simulink library "bcm"  (R2021b)
settings: Solver=VariableStepAuto  StartTime=0.0  StopTime=10.0  RelTol=1e-3
undefined symbols (not defined in the file or in its folder): ENUM_ANTITHEFT_ALARM, ENUM_ANTITHEFT_ARM, ENUM_ANTITHEFT_DISARM, ENUM_ANTITHEFT_WAIT, ENUM_GEARPOSNTOCAN_P, ENUM_PDKEYRAWLULOCK_INUNLOCK, ENUM_PDKEYRAWPS_INPS, ENUM_POWERSTA_ON, ENUM_POWERSTA_READY, ENUM_POWERSTA_STANDBY, FALSE, KBCM_ALMBrightnessDark_enum, KBCM_AmbBlue_enum, KBCM_AmbBreathT_ms, KBCM_AmbGreen_enum, KBCM_AmbRed_enum, KBCM_Antitheft_enum_ovrdflg, KBCM_Antitheft_enum_ovrdval, KBCM_APMDoorCtrlSta_flg_ovrdflg, KBCM_APMDoorCtrlSta_flg_ovrdval, KBCM_DelayTSW_flg, KBCM_DiagFLTC_mA, KBCM_DiagFMHT_s, KBCM_DiagFRTC_mA, KBCM_DiagRLTC_mA, KBCM_DiagRRTC_mA, KBCM_DrAPMRetryTimes_cnt, KBCM_DrOpenWdwOT_s, KBCM_DrOpenWdwReady_s, KBCM_ESSOffT_ms, KBCM_ESSOnT_ms, KBCM_IVIRstHoldT_ms, KBCM_IVIRstTriggerT_ms, KBCM_ONDelayT_ms, KBCM_ReDetectT_K, KBCM_RmLampKeep_min, KBCM_RmLpKeyInT_s, KBCM_RmLpKeyMissT_s, KBCM_SlpDebounceTime_s, KBCM_SPTGDetectT_sec, KBCM_SPTGLeave_flg, KBCM_SPTGLeftBound_cm, KBCM_SPTGLeftBoundOut_cm, KBCM_SPTGLowerBound_cm, KBCM_SPTGLowerBoundOut_cm, KBCM_SPTGRightBound_cm, KBCM_SPTGRightBoundOut_cm, KBCM_SPTGTOut_K, KBCM_SPTGUpperBound_cm, KBCM_SPTGUpperBoundOut_cm, KBCM_SPTGWaitDKC_sec, KBCM_TrunSWKeepTime3_s, KBCM_TrunSWKeepTime5_s, KBCM_TrunSWKeepTime7_s, KBCM_USSDis_cm, KBCM_USSFilterT_K, KBCM_WaitAPMPwr_K, KBCM_WdwManualDetT_s, MIN2SEC, TRUE ... (+1)
libraries: simulink x151, hcu_lib x5
(part 2 of 8)

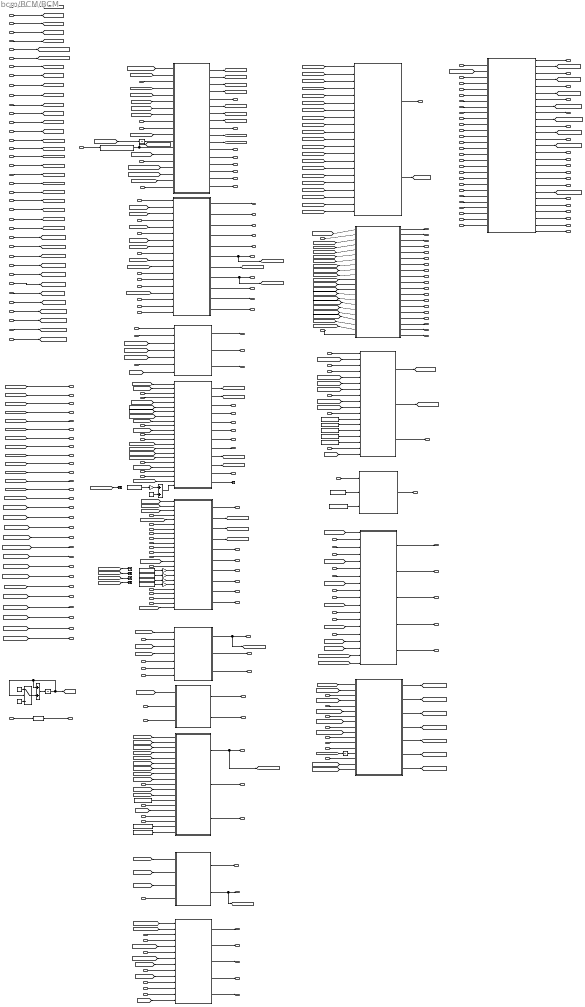
== system bcm/BCM/BCM ==
  task_time_s : Inport
  VINP_VehSpeed_kph : Inport  Port=2
  VINP_AirBagFailCmd_flg : Inport  Port=3
  VINP_ActBrkLampSta_flg : Inport  Port=4
  VINP_ESSActive_flg : Inport  Port=5
  VINP_SASAngle_Deg : Inport  Port=6
  VINP_SRRODAWarnR_enum : Inport  Port=7
  VINP_SRRODAWarnL_enum : Inport  Port=8
  VINP_SRRBSDWarnR_enum : Inport  Port=9
  VINP_SRRBSDWarnL_enum : Inport  Port=10
  VINP_LeftTurnReq_flg : Inport  Port=11
  VINP_RightTurnReq_flg : Inport  Port=12
  VINP_ForceLowBeam_enum : Inport  Port=13
  VINP_HazardWarningReq_flg : Inport  Port=14
  VINP_SetUnlockSingle_flg : Inport  Port=15
  VINP_IVIStatus_flg : Inport  Port=16
  VINP_IVINightModeSta_flg : Inport  Port=17
  VINP_HeadLampSW_enum : Inport  Port=18
  VINP_RFogLampSW_flg : Inport  Port=19
  VINP_FollowMeSW_flg : Inport  Port=20
  VINP_IVIRRDefReq_flg : Inport  Port=21
  VINP_IVIWIMAINSW_flg : Inport  Port=22
  VINP_CANMsgValidIVI2_flg : Inport  Port=23
  VINP_CDLUnlockButt_flg : Inport  Port=24  OutDataTypeStr=boolean
  VINP_CDLLockButt_flg : Inport  Port=25  OutDataTypeStr=boolean
  VINP_RoomLampMode_flg : Inport  Port=26
  VINP_MFRDNBrightReq_pct : Inport  Port=27
  VINP_METERKPHCalcu_kph : Inport  Port=28
  VINP_IVIPWModeReq_enum : Inport  Port=29
  VINP_AmbLighLowBatAlertSW_flg : Inport  Port=30
  VINP_AmbLighSafetyAlertSW_flg : Inport  Port=31
  VINP_AmbLightBrightnessSet_enum : Inport  Port=32
  VINP_AmbLightDimInDarkSW_flg : Inport  Port=33
  VINP_AmbLightSW_flg : Inport  Port=34
  VINP_AmbLightWlcmLightSW_flg : Inport  Port=35
  VINP_LINKtoDRIVE_flg : Inport  Port=36
  VINP_AmbLightColorSet_enum : Inport  Port=37
  VINP_IVIPTGUSStaSW_flg : Inport  Port=38
  VINP_LDrvControlCommand_pct : Inport  Port=39
  VINP_LPasControlCommand_pct : Inport  Port=40
  VINP_LRLDControlCommand_pct : Inport  Port=41
  VINP_LRRDControlCommand_pct : Inport  Port=42
  VINP_OpenDrOpenWdoSW_flg : Inport  Port=43
  VINP_CANMsgValidIVI1_flg : Inport  Port=44
  VINP_UserSet_enum : Inport  Port=45
  VINP_TurnSwTimeSet_enum : Inport  Port=46
  VINP_IVILockSoundSWSta_flg : Inport  Port=47
  VINP_AVMparkingmode_enum : Inport  Port=48
  VINP_HVBattSOCDis_pct : Inport  Port=49
  VINP_CSW2DimSwSta_flg : Inport  Port=50
  VINP_CSW2PassSWSta_flg : Inport  Port=51
  VINP_CSW2FWipSwSta_enum : Inport  Port=52
  VINP_CSW2FWasSwSta_enum : Inport  Port=53
  VUNP_CSW2TurnSwSta_enum : Inport  Port=54
  VINP_CSW2RWipWasSwSta_enum : Inport  Port=55
  VINP_PCommandToBCM_enum : Inport  Port=56
  VINP_DrLockSta_flg : Inport  Port=57
  VINP_CSWDimSw_flg : Inport  Port=58
  VINP_CSWPassSWSta_flg : Inport  Port=59
  VINP_RLSLampSta_flg : Inport  Port=60
  VINP_CSWTurnSWSta_enum : Inport  Port=61
  VINP_RLTurnLampC_mA : Inport  Port=62
  VINP_RRTurnLampC_mA : Inport  Port=63
  VINP_FLTurnLampC_mA : Inport  Port=64
  VINP_FRTurnLampC_mA : Inport  Port=65
  VINP_MIRRORFOLDSW_flg : Inport  Port=66
  VINP_CSWFWasSWSta_enum : Inport  Port=67
  VINP_CSWFWipSWSta_enum : Inport  Port=68
  VINP_RLSRainSnrWiperCmd_enum : Inport  Port=69
  VINP_FWiperAS_flg : Inport  Port=70
  VINP_CSWRWipIntSwSta_enum : Inport  Port=71
  VINP_RWiperAS_flg : Inport  Port=72
  VINP_CSWRWasSWSta_enum : Inport  Port=73
  VINP_PTGRDILsta_enum : Inport  Port=74
  VINP_RWiperProtection_flg : Inport  Port=75
  VINP_FWiperProtection_flg : Inport  Port=76
  VINP_PDKeyAreaPTG_enum : Inport  Port=77
  VINP_SWCmodeSta_flg : Inport  Port=78
  VINP_CANMsgValidDKC1_flg : Inport  Port=79
  VINP_CANMsgValidGWZoneDR1_flg : Inport  Port=80
  VINP_CANMsgValidGWZoneFR1_flg : Inport  Port=81
  VINP_PTGInnerSW2_enum : Inport  Port=82
  VINP_LDrvValWdwOpened_pct : Inport  Port=83
  VINP_LPasValWdwOpened_pct : Inport  Port=84
  VINP_LRLDValWdwOpened_pct : Inport  Port=85
  VINP_LRRDValWdwOpened_pct : Inport  Port=86
  VINP_PDKeyAreaLockUnlock_enum : Inport  Port=87
  VINP_PDKeyAreaPS_enum : Inport  Port=88
  VINP_ReDoorLock_enum : Inport  Port=89
  VINP_ReOutsideMirror_enum : Inport  Port=90
  VINP_HoodSW_flg : Inport  Port=91
  VINP_TailgateSW_flg : Inport  Port=92
  VINP_DrDoorSW_flg : Inport  Port=93
  VINP_PsDoorSW_flg : Inport  Port=94
  VINP_RLDoorSW_flg : Inport  Port=95
  VINP_RRDoorSW_flg : Inport  Port=96
  VINP_TrunkHanSW_flg : Inport  Port=97
  VINP_HazardSW_flg : Inport  Port=98
  VINP_CentralDoorLockSW_flg : Inport  Port=99
  VINP_BrakeSWGPIO_flg : Inport  Port=100
  VPMM_PwrSta_enum : Inport  Port=101
  VTQD_ShiftGearPosn_enum : Inport  Port=102
  VTQD_CrashDetd_flg : Inport  Port=103
  VTQD_DiagHCrash_flg : Inport  Port=104
  VTQD_ReBrakeLPReq_flg : Inport  Port=105
  VINP_FlashAntitheft_enum : Inport  Port=106
  VINP_FlashCountAlarm_enum : Inport  Port=107
  VINP_FlashMFSWTri_flg : Inport  Port=108
  VINP_FlashMirrorFlodPos : Inport  Port=109
  VINP_FlashFuelDoorPos : Inport  Port=110
  VINP_FlashLockSetting_flg : Inport  Port=111
  VINP_FlashMFRDNBrightReq_pct : Inport  Port=112
  VINP_FlashRoomLampMode_flg : Inport  Port=113
  VINP_FlashWiperFixMode_flg : Inport  Port=114
  VINP_FlashIVIPTGUSStaSW_flg : Inport  Port=115
  VINP_FlashHoodSW_flg : Inport  Port=116
  VINP_FlashTailgateSW_flg : Inport  Port=117
  VINP_FlashCTDLockSW_flg : Inport  Port=118
  VINP_FlashTailgateHDSW_flg : Inport  Port=119
  VINP_FlashAPMDoorControlSta_flg : Inport  Port=120
  VINP_FlashfUnlockSingle_flg : Inport  Port=121
  VINP_FlashAmbFunEN_enum : Inport  Port=122
  VINP_FlashAmbWelEN_enum : Inport  Port=123
  VINP_FlashAmbDimEN_enum : Inport  Port=124
  VINP_FlashAmbLinkDriSta_enum : Inport  Port=125
  VINP_FlashAmbPwrWarnEN_enum : Inport  Port=126
  VINP_FlashAmbODAEN_enum : Inport  Port=127
  VINP_FlashAmbColorSta1_enum : Inport  Port=128
  VINP_FlashAmbColorSta2_enum : Inport  Port=129
  VINP_FlashAmbColorSta3_enum : Inport  Port=130
  VINP_FlashAmbColorSta4_enum : Inport  Port=131
  VINP_FlashAmbColorSta5_enum : Inport  Port=132
  VINP_FlashAmbColorSta7_enum : Inport  Port=133
  VINP_FlashAmbBrightnessSta1_enum : Inport  Port=134
  VINP_FlashAmbBrightnessSta2_enum : Inport  Port=135
  VINP_FlashAmbBrightnessSta3_enum : Inport  Port=136
  VINP_FlashAmbBrightnessSta4_enum : Inport  Port=137
  VINP_FlashAmbBrightnessSta5_enum : Inport  Port=138
  VINP_FlashAmbBrightnessSta7_enum : Inport  Port=139
  VINP_funAuto_flg : Inport  Port=140
  VINP_DiagDRLOFF_flg : Inport  Port=141
  VINP_DiagFMHT_s : Inport  Port=142
  VINP_DiagFLTC_mA : Inport  Port=143
  VINP_DiagFRTC_mA : Inport  Port=144
  VINP_DiagRLTC_mA : Inport  Port=145
  VINP_DiagRRTC_mA : Inport  Port=146
  VAPM_PASDRMR_cm : Inport  Port=147
  VAPM_PASDRML_cm : Inport  Port=148
  VINP_APSActive_flg : Inport  Port=149
  VINP_RRDefSta_flg : Inport  Port=150
  VDDM_HVRlyOpCFS_flg : Inport  Port=151
  VDDM_MCUActCFS_flg : Inport  Port=152
  APM_Door : Subsystem
  Add1 : Sum
  Amb : Subsystem
  AntiTheft : Subsystem
  BCM_WAKE_MODULE : Subsystem
  CSW : Subsystem
  CenterDoorLock : Subsystem
  Constant10 : Constant  Value=KBCM_DelayTSW_flg
  Constant11 : Constant  Value=KBCM_ReDetectT_K
  Constant12 : Constant  Value=KBCM_SPTGDetectT_sec
  Constant13 : Constant  Value=KBCM_SPTGLeave_flg
  Constant14 : Constant  Value=KBCM_RmLampKeep_min
  Constant15 : Constant  Value=KBCM_SPTGWaitDKC_sec
  Constant16 : Constant  Value=0
  Constant17 : Constant
  Constant18 : Constant  Value=KBCM_RmLpKeyInT_s
  Constant19 : Constant  Value=KBCM_RmLpKeyMissT_s
  Constant44 : Constant  Value=KBCM_DiagFMHT_s
  Constant45 : Constant  Value=10
  Constant46 : Constant  Value=KBCM_DiagFLTC_mA
  Constant47 : Constant  Value=KBCM_DiagFRTC_mA
  Constant48 : Constant  Value=KBCM_DiagRLTC_mA
  Constant49 : Constant  Value=KBCM_DiagRRTC_mA
  Constant8 : Constant  Value=KBCM_IVIRstHoldT_ms
  Constant9 : Constant  Value=KBCM_IVIRstTriggerT_ms
  Data Type Conversion : DataTypeConversion  OutDataTypeStr=uint8
  Dimmer : Subsystem
  ExteriorLight : Subsystem
  FlasherSignal : Subsystem
  Gain{,2..4} (4 alike) : Gain  Gain=10
  Gain1 : Gain  Gain=5
  IVI Reset : Subsystem
  PTG : Subsystem
  Personal_Setting : Subsystem
  PowerMirror : Subsystem
  RearDefogger : Subsystem
  RoomLamp : Subsystem
  Sum : Sum
  Switch : Switch  Criteria=u2 > Threshold
  Tailgate : Subsystem
  Terminator{,1..5} (6 alike) : Terminator
  Unit Delay : UnitDelay  SampleTime=-1  HasFrameUpgradeWarning=on
  Unit Delay1 : UnitDelay  SampleTime=-1  HasFrameUpgradeWarning=on
  Unit Delay2 : UnitDelay  SampleTime=-1  HasFrameUpgradeWarning=on
  Verify : Subsystem
  WasherWiper : Subsystem
  VBCM_AntitheftSta_enum : Outport
  VBCM_TailgateRemote_enum : Outport  Port=2
  VBCM_HornCtrl_flg : Outport  Port=3
  VBCM_AllDoorSW_flg : Outport  Port=4
  VBCM_BCMDoorLockSta_flg : Outport  Port=5
  VBCM_AntitheftSeatFlod_flg : Outport  Port=6
  VBCM_HoodSW_flg : Outport  Port=7
  VBCM_TailgateSW_flg : Outport  Port=8
  VBCM_DrDoorSW_flg : Outport  Port=9
  VBCM_PsDoorSW_flg : Outport  Port=10
  VBCM_RLDoorSW_flg : Outport  Port=11
  VBCM_RRDoorSW_flg : Outport  Port=12
  VBCM_LockSetting_flg : Outport  Port=13
  VBCM_FrChargingDoorCtrl_enum : Outport  Port=14
  VBCM_RrChargingDoorCtrl_enum : Outport  Port=15
  VBCM_CrashSDetd_flg : Outport  Port=16
  VBCM_CTDCtrl_enum : Outport  Port=17
  VBCM_DoorLockIND_flg : Outport  Port=18
  VBCM_CTDLockSW_flg : Outport  Port=19
  VBCM_Dimmer_pct : Outport  Port=20
  VBCM_DimmerEN_flg : Outport  Port=21
  VBCM_PosLamp_flg : Outport  Port=22
  VBCM_LBeam_flg : Outport  Port=23
  VBCM_HBeam_flg : Outport  Port=24
  VBCM_RrFogLamp_flg : Outport  Port=25
  VBCM_BrakeLamp_flg : Outport  Port=26
  VBCM_ReverseLamp_flg : Outport  Port=27
  VBCM_LDRL_flg : Outport  Port=28
  VBCM_RDRL_flg : Outport  Port=29
  VBCM_LBSD_flg : Outport  Port=30
  VBCM_RBSD_flg : Outport  Port=31
  VBCM_HazardSW_flg : Outport  Port=32
  VBCM_LTurnLP_flg : Outport  Port=33
  VBCM_RTurnLP_flg : Outport  Port=34
  VBCM_BCMBuzzerReq_flg : Outport  Port=35
  VBCM_MirrorCtrl_enum : Outport  Port=36
  VBCM_MirrorDefog_flg : Outport  Port=37
  VBCM_RrDefog_flg : Outport  Port=38
  VBCM_RoomLampH_flg : Outport  Port=39
  VBCM_RoomLampL_flg : Outport  Port=40
  VBCM_TrunkRel_flg : Outport  Port=41
  VBCM_TailgateHDSW_flg : Outport  Port=42
  VBCM_FWiperL_flg : Outport  Port=43
  VBCM_FWiperH_flg : Outport  Port=44
  VBCM_RWiper_flg : Outport  Port=45
  VBCM_WasherCtrl_enum : Outport  Port=46
  VBCM_WiperFixMode_flg : Outport  Port=47
  VBCM_SleepReq_flg : Outport  Port=48
  VBCM_AmbLightBreath1_enum : Outport  Port=49
  VBCM_AmbLightBreath2_enum : Outport  Port=50
  VBCM_AmbLightBreath3_enum : Outport  Port=51
  VBCM_AmbLightBreath4_enum : Outport  Port=52
  VBCM_AmbLightBreath5_enum : Outport  Port=53
  VBCM_AmbLightBreath6_enum : Outport  Port=54
  VBCM_AmbLightBrightness1_enum : Outport  Port=55
  VBCM_AmbLightBrightness2_enum : Outport  Port=56
  VBCM_AmbLightBrightness3_enum : Outport  Port=57
  VBCM_AmbLightBrightness4_enum : Outport  Port=58
  VBCM_AmbLightBrightness5_enum : Outport  Port=59
  VBCM_AmbLightBrightness6_enum : Outport  Port=60
  VBCM_AmbLightColor1_enum : Outport  Port=61
  VBCM_AmbLightColor2_enum : Outport  Port=62
  VBCM_AmbLightColor3_enum : Outport  Port=63
  VBCM_AmbLightColor4_enum : Outport  Port=64
  VBCM_AmbLightColor5_enum : Outport  Port=65
  VBCM_AmbLightColor6_enum : Outport  Port=66
  VBCM_LampPwr_flg : Outport  Port=67
  VBCM_SPTGDet_flg : Outport  Port=68
  VBCM_APSOpenPTG_flg : Outport  Port=69
  VBCM_FollowMe_flg : Outport  Port=70
  VBCM_IVIRST_flg : Outport  Port=71
  VBCM_CountAlarm_enum : Outport  Port=72
  VBCM_MFSWTri_flg : Outport  Port=73
  VBCM_MirrorFlodPos_flg : Outport  Port=74
  VBCM_FuelDoorPos_flg : Outport  Port=75
  VBCM_MFRDNBrightReq_pct : Outport  Port=76
  VBCM_RoomLampMode_flg : Outport  Port=77
  VBCM_IVIPTGUSStaSW_flg : Outport  Port=78
  VBCM_PTGInnerSW2_enum : Outport  Port=79
  VBCM_DiagHCrash_flg : Outport  Port=80
  VBCM_DiagFLTS_flg : Outport  Port=81
  VBCM_DiagFRTS_flg : Outport  Port=82
  VBCM_DiagRLTS_flg : Outport  Port=83
  VBCM_DiagRRTS_flg : Outport  Port=84
  VBCM_LDrvCtrlCmd_pct : Outport  Port=85
  VBCM_LPasCtrlCmd_pct : Outport  Port=86
  VBCM_LRLDCtrlCmd_pct : Outport  Port=87
  VBCM_LRRDCtrlCmd_pct : Outport  Port=88
  VBCM_APMDoorControlSta_flg : Outport  Port=89
  VBCM_AmbFunEN_flg : Outport  Port=90
  VBCM_AmbWelEN_flg : Outport  Port=91
  VBCM_AmbDimEN_flg : Outport  Port=92
  VBCM_AmbLinkDriSta_flg : Outport  Port=93
  VBCM_AmbPwrWarnEN_flg : Outport  Port=94
  VBCM_AmbODAEN_flg : Outport  Port=95
  VBCM_AmbColorSta_enum : Outport  Port=96
  VBCM_AmbBrightSta_enum : Outport  Port=97
  VBCM_LockAlarm_enum : Outport  Port=98
  VBCM_ATCtrl_enum : Outport  Port=99
  VBCM_fUnlockSingle_flg : Outport  Port=100
  VBCM_UserNow_enum : Outport  Port=101
  VBCM_AmbFunENFlash_enum : Outport  Port=102
  VBCM_AmbWelENFlash_enum : Outport  Port=103
  VBCM_AmbDimENFlash_enum : Outport  Port=104
  VBCM_AmbLinkDriStaFlash_enum : Outport  Port=105
  VBCM_AmbPwrWarnENFlash_enum : Outport  Port=106
  VBCM_AmbODAENFlash_enum : Outport  Port=107
  VBCM_AmbColorSta1_enum : Outport  Port=108
  VBCM_AmbColorSta2_enum : Outport  Port=109
  VBCM_AmbColorSta3_enum : Outport  Port=110
  VBCM_AmbColorSta4_enum : Outport  Port=111
  VBCM_AmbColorSta5_enum : Outport  Port=112
  VBCM_AmbColorSta7_enum : Outport  Port=113
  VBCM_AmbBrightnessSta1_enum : Outport  Port=114
  VBCM_AmbBrightnessSta2_enum : Outport  Port=115
  VBCM_AmbBrightnessSta3_enum : Outport  Port=116
  VBCM_AmbBrightnessSta4_enum : Outport  Port=117
  VBCM_AmbBrightnessSta5_enum : Outport  Port=118
  VBCM_AmbBrightnessSta7_enum : Outport  Port=119
  VBCM_HazardIND_flg : Outport  Port=120
  VBCM_DimSwSta_flg : Outport  Port=121
  VBCM_PassSWSta_flg : Outport  Port=122
  VBCM_FWipSwSta_enum : Outport  Port=123
  VBCM_FWasSwSta_enum : Outport  Port=124
  VBCM_TurnSwSta_enum : Outport  Port=125
  wires:
  VPMM_PwrSta_enum/1 -> [VPMM_PwrSta_enum]
  VINP_HoodSW_flg/1 -> AntiTheft/3(VINP_HoodSW_flg)
  VINP_TailgateSW_flg/1 -> [VINP_TailgateSW_flg]
  VINP_DrLockSta_flg/1 -> AntiTheft/9(VINP_DrLockSta_flg)
  VINP_ReDoorLock_enum/1 -> AntiTheft/10(VINP_ReDoorLock_enum)
  VINP_VehSpeed_kph/1 -> [VINP_VehSpeed_kph]
  AntiTheft/4(VBCM_AntitheftSta_enum) -> [VBCM_AntitheftSta_enum]
  AntiTheft/5(VBCM_TailgateRemote_enum) -> VBCM_TailgateRemote_enum/1
  AntiTheft/6(VBCM_HornCtrl_flg) -> [VBCM_HornCtrl_flg]
  AntiTheft/7(VBCM_AllDoorSW_flg) -> [VBCM_AllDoorSW_flg]
  AntiTheft/9(VBCM_AntitehftSeatFlod_flg) -> VBCM_AntitheftSeatFlod_flg/1
  AntiTheft/8(VBCM_BCMDoorLockSta_flg) -> [VBCM_BCMDoorLockSta_flg]
  AntiTheft/1(VBCM_ATCtrl_enum) -> [VBCM_ATCtrl_enum]
  AntiTheft/2(VBCM_ATActCtrl_enum) -> [VBCM_ATActCtrl_enum]
  AntiTheft/3(VBCM_ATAlarm_flg) -> [VBCM_ATAlarm_flg]
  [VBCM_AllDoorSW_flg] -> CenterDoorLock/3(VBCM_AllDoorSW_flg)
  [VBCM_AntitheftSta_enum] -> CenterDoorLock/2(VBCM_AntitheftSta_enum)
  [VPMM_PwrSta_enum] -> CenterDoorLock/5(VPMM_PwrSta_enum)
  CenterDoorLock/1(VBCM_LockSetting_flg) -> VBCM_LockSetting_flg/1
  CenterDoorLock/7(VBCM_fVIGHandle_flg) -> [VBCM_fVIGHandle_flg]
  VTQD_DiagHCrash_flg/1 -> CenterDoorLock/4(VTQD_DiagHCrash_flg)
  VINP_SetUnlockSingle_flg/1 -> CenterDoorLock/1(VINP_SetUnlockSingle_flg)
  VINP_CentralDoorLockSW_flg/1 -> CenterDoorLock/6(VINP_CentralDoorLockSW_flg)
  [VBCM_BCMDoorLockSta_flg] -> CenterDoorLock/7(VBCM_BCMDoorLockSta_flg)
  [VBCM_ATActCtrl_enum] -> CenterDoorLock/8(VBCM_ATActCtrl_enum)
  [VINP_VehSpeed_kph] -> CenterDoorLock/10(VINP_VehSpeed_kph)
  VINP_AirBagFailCmd_flg/1 -> CenterDoorLock/9(VINP_AirBagFailCmd_flg)
  CenterDoorLock/2(VBCM_FrChargingDoorCtrl_enum) -> VBCM_FrChargingDoorCtrl_enum/1
  CenterDoorLock/3(VBCM_RrChargingDoorCtrl_enum) -> VBCM_RrChargingDoorCtrl_enum/1
  CenterDoorLock/4(VBCM_CrashDetd_flg) -> VBCM_CrashSDetd_flg/1
  CenterDoorLock/5(VBCM_CTDCtrl_enum) -> VBCM_CTDCtrl_enum/1
  CenterDoorLock/6(DoorLockIND) -> [VBCM_DoorLockIND_flg], VBCM_DoorLockIND_flg/1
  VINP_MFRDNBrightReq_pct/1 -> Dimmer/1(VINP_MFRDNBrightReq_pct)
  VINP_IVIStatus_flg/1 -> Dimmer/2(VINP_IVIStatus_flg)
  Dimmer/1(VBCM_Dimmer_pct) -> VBCM_Dimmer_pct/1
  Dimmer/2(VBCM_DimmerEN_flg) -> VBCM_DimmerEN_flg/1
  [VBCM_PosLamp_flg] -> Dimmer/4(VBCM_PosLamp_flag)
  [VPMM_PwrSta_enum] -> PowerMirror/1(VPMM_PwrSta_enum)
  VINP_MIRRORFOLDSW_flg/1 -> PowerMirror/2(VINP_MIRRORFOLDSW_flg)
  [VINP_VehSpeed_kph] -> PowerMirror/3(VINP_VehSpeed_kph)
  [VBCM_ATActCtrl_enum] -> PowerMirror/4(VBCM_ATActCtrl_enum)
  PowerMirror/1(VBCM_MirrorCtrl_enum) -> [VBCM_MirrorCtrl_enum], VBCM_MirrorCtrl_enum/1
  [VPMM_PwrSta_enum] -> RearDefogger/1(VPMM_PwrSta_enum)
  VINP_RRDefSta_flg/1 -> RearDefogger/2(VINP_RRDefSta_flg)
  VINP_IVIRRDefReq_flg/1 -> RearDefogger/3(VINP_IVIRRDefReq_flg)
  RearDefogger/1(VBCM_MirrorDefog_flg) -> VBCM_MirrorDefog_flg/1
  RearDefogger/2(VBCM_RrDefog_flg) -> VBCM_RrDefog_flg/1
  [VPMM_PwrSta_enum] -> RoomLamp/2(VPMM_PwrSta_enum)
  [VBCM_BCMDoorLockSta_flg] -> RoomLamp/3(VBCM_BCMDoorLockSta_flg)
  [VBCM_AllDoorSW_flg] -> RoomLamp/4(VBCM_AllDoorSW_flg)
  [VBCM_AntitheftSta_enum] -> RoomLamp/5(VBCM_AntitheftSta_enum)
  [VPMM_PwrSta_enum] -> Tailgate/1(VPMM_PwrSta_enum)
  [VINP_VehSpeed_kph] -> Tailgate/2(VINP_VehSpeed_kph)
  [VBCM_BCMDoorLockSta_flg] -> Tailgate/3(VBCM_BCMDoorLockSta_flg)
  VINP_TrunkHanSW_flg/1 -> Tailgate/4(VINP_TrunkHandleSwSG08_flg)
  Tailgate/1(VBCM_TrunkRel_flg) -> VBCM_TrunkRel_flg/1
  Unit Delay/1 -> AntiTheft/12(VBCM_fVIGHandle_flg)
  [VBCM_fVIGHandle_flg] -> Unit Delay/1
  VINP_CDLUnlockButt_flg/1 -> CenterDoorLock/12(VINP_CDLUnlockButt_flg)
  VINP_CDLLockButt_flg/1 -> CenterDoorLock/13(VINP_CDLLockButt_flg)
  VTQD_CrashDetd_flg/1 -> CenterDoorLock/14(VTQD_CrashDetd_flg)
  VINP_RoomLampMode_flg/1 -> RoomLamp/10(VINP_RoomLampMode_flg)
  AntiTheft/10(VBCM_HoodSW_flg) -> [VBCM_HoodSW_flg]
  AntiTheft/11(VBCM_TailgateSW_flg) -> [VBCM_TailgateSW_flg]
  AntiTheft/12(VBCM_DrDoorSW_flg) -> VBCM_DrDoorSW_flg/1
  AntiTheft/13(VBCM_PsDoorSW_flg) -> VBCM_PsDoorSW_flg/1
  AntiTheft/14(VBCM_RLDoorSW_flg) -> VBCM_RLDoorSW_flg/1
  AntiTheft/15(VBCM_RRDoorSW_flg) -> VBCM_RRDoorSW_flg/1
  CenterDoorLock/8(VBCM_CTDLockSW_flg) -> [VBCM_CTDLockSW_flg], VBCM_CTDLockSW_flg/1
  Tailgate/2(VBCM_TailgateHDSW_flg) -> [VBCM_TailgateHDSW_flg], VBCM_TailgateHDSW_flg/1
  VINP_CANMsgValidIVI2_flg/1 -> [VINP_CANMsgValidIVI2_flg]
  [VINP_CANMsgValidIVI2_flg] -> RoomLamp/11(VINP_CANMsgValidIVI2_flg)
  [VINP_TailgateSW_flg] -> RoomLamp/12(VINP_TailgateSW_flg)
  [VINP_CANMsgValidIVI2_flg] -> CenterDoorLock/15(VINP_CANMsgValidIVI2_flg)
  CenterDoorLock/10(VBCM_DiagHCrash_flg) -> VBCM_DiagHCrash_flg/1
  [VBCM_ATCtrl_enum] -> FlasherSignal/1(VBCM_ATCtrl_enum)
  [VBCM_ATAlarm_flg] -> FlasherSignal/2(VBCM_ATAlarm_flg)
  [VPMM_PwrSta_enum] -> FlasherSignal/3(VPMM_PwrSta_enum)
  VINP_HazardSW_flg/1 -> FlasherSignal/4(VINP_HazardSW_flg)
  VINP_RLTurnLampC_mA/1 -> FlasherSignal/6(VINP_RLTurnLampC_mA)
  VINP_RRTurnLampC_mA/1 -> FlasherSignal/7(VINP_RRTurnLampC_mA)
  VINP_FLTurnLampC_mA/1 -> FlasherSignal/8(VINP_FLTurnLampC_mA)
  VINP_FRTurnLampC_mA/1 -> FlasherSignal/9(VINP_FRTurnLampC_mA)
  VINP_PTGRDILsta_enum/1 -> FlasherSignal/10(VINP_PTGRDILsta_enum)
  VINP_ESSActive_flg/1 -> FlasherSignal/11(VINP_ESSActive_flg)
  VINP_LeftTurnReq_flg/1 -> FlasherSignal/12(VINP_LeftTurnReq_flg)
  VINP_RightTurnReq_flg/1 -> FlasherSignal/13(VINP_RightTurnReq_flg)
  VINP_HazardWarningReq_flg/1 -> FlasherSignal/15(HazardWarningReq)
  FlasherSignal/1(VBCM_HazardSW_flg) -> VBCM_HazardSW_flg/1
  FlasherSignal/2(VBCM_LTurnLP_flg) -> [VBCM_LTurnLP_flg]
  task_time_s/1 -> [task_time_s]
  [VBCM_HoodSW_flg] -> BCM_WAKE_MODULE/1(VBCM_HoodSW_flg)
  [VBCM_TailgateSW_flg] -> BCM_WAKE_MODULE/2(VBCM_TailgateSW_flg)
  [VBCM_CTDLockSW_flg] -> BCM_WAKE_MODULE/3(VBCM_CTDLockSW_flg)
  [VBCM_TailgateHDSW_flg] -> BCM_WAKE_MODULE/4(VBCM_TailgateHDSW_flg)
  [VBCM_AntitheftSta_enum] -> BCM_WAKE_MODULE/5(VBCM_AntitheftSta_enum)
  [VBCM_AllDoorSW_flg] -> BCM_WAKE_MODULE/6(VBCM_AllDoorSW_flg)
  [VBCM_HornCtrl_flg] -> BCM_WAKE_MODULE/7(VBCM_HornCtrl_flg)
  [VBCM_DoorLockIND_flg] -> BCM_WAKE_MODULE/8(VBCM_DoorLockIND_flg)
  [VINP_BrakeSWGPIO_flg] -> BCM_WAKE_MODULE/9(VINP_BrakeSWGPIO_flg)
  [VBCM_PosLamp_flg] -> BCM_WAKE_MODULE/10(VBCM_PosLamp_flg)
  [VBCM_LBSD_flg] -> BCM_WAKE_MODULE/11(VBCM_LBSD_flg)
  [VBCM_RBSD_flg] -> BCM_WAKE_MODULE/12(VBCM_RBSD_flg)
  [VBCM_RTurnLP_flg] -> BCM_WAKE_MODULE/14(VBCM_RTurnLP_flg)
  [VBCM_LTurnLP_flg] -> BCM_WAKE_MODULE/13(VBCM_LTurnLP_flg)
  [VBCM_MirrorCtrl_enum] -> BCM_WAKE_MODULE/15(VBCM_MirrorCtrl_enum)
  [VBCM_RoomLampH_flg] -> BCM_WAKE_MODULE/16(VBCM_RoomLampH_flg)
  [task_time_s] -> BCM_WAKE_MODULE/17(task_time_s)
  BCM_WAKE_MODULE/1(VBCM_SleepReq_flg) -> VBCM_SleepReq_flg/1
  [VPMM_PwrSta_enum] -> ExteriorLight/2(VPMM_PwrSta_enum)
  VINP_ForceLowBeam_enum/1 -> ExteriorLight/18(VINP_ForceLowBeam_enum)
  VTQD_ReBrakeLPReq_flg/1 -> ExteriorLight/20(VTQD_ReBrakeLPReq_flg)
  VINP_METERKPHCalcu_kph/1 -> ExteriorLight/21(VINP_METERKPHCalcu_kph)
  VINP_SRRBSDWarnR_enum/1 -> [VINP_SRRBSDWarnR_enum]
  VINP_SRRODAWarnL_enum/1 -> [VINP_SRRODAWarnL_enum]
  VINP_SRRODAWarnR_enum/1 -> [VINP_SRRODAWarnR_enum]
  VINP_ActBrkLampSta_flg/1 -> ExteriorLight/13(VINP_ActBrkLampSta_flg)
  VINP_RLSLampSta_flg/1 -> ExteriorLight/12(VINP_RLSLampSta_flg)
  VINP_FollowMeSW_flg/1 -> ExteriorLight/10(VINP_FollowMeSW_flg)
  VINP_RFogLampSW_flg/1 -> ExteriorLight/4(VINP_RFogLampSW_flg)
  VINP_HeadLampSW_enum/1 -> ExteriorLight/3(VINP_HeadLampSW_enum)
  [VINP_CANMsgValidIVI2_flg] -> ExteriorLight/19(VINP_CANMsgValidIVI2_flg)
  [VBCM_ATCtrl_enum] -> ExteriorLight/11(VBCM_ATCtrl_enum)
  [VBCM_OutMode_enum] -> ExteriorLight/9(VBCM_OutMode_enum)
  VINP_BrakeSWGPIO_flg/1 -> [VINP_BrakeSWGPIO_flg]
  [VINP_BrakeSWGPIO_flg] -> ExteriorLight/5(VINP_BrakeSWGPIO_flg)
  ExteriorLight/3(VBCM_HBeam_flg) -> VBCM_HBeam_flg/1
  ExteriorLight/1(VBCM_PosLamp_flg) -> [VBCM_PosLamp_flg]
  ExteriorLight/4(VBCM_RrFogLamp_flg) -> VBCM_RrFogLamp_flg/1
  ExteriorLight/5(VBCM_BrakeLamp_flg) -> VBCM_BrakeLamp_flg/1
  ExteriorLight/6(VBCM_ReverseLamp_flg) -> VBCM_ReverseLamp_flg/1
  ExteriorLight/7(VBCM_LDRL_flg) -> VBCM_LDRL_flg/1
  ExteriorLight/8(VBCM_RDRL_flg) -> VBCM_RDRL_flg/1
  ExteriorLight/10(VBCM_RBSD_flg) -> [VBCM_RBSD_flg]
  ExteriorLight/9(VBCM_LBSD_flg) -> [VBCM_LBSD_flg]
  ExteriorLight/12(VBCM_showup_flg) -> Terminator5/1
  [VINP_TailgateSW_flg] -> AntiTheft/4(VINP_TailgateSW_flg)
  [VINP_DrDoorSW_flg] -> AntiTheft/5(VINP_DrDoorSW_flg)
  [VINP_VehSpeed_kph] -> AntiTheft/11(VINP_VehSpeed_kph)
  VINP_DrDoorSW_flg/1 -> [VINP_DrDoorSW_flg]
  [VPMM_PwrSta_enum] -> AntiTheft/2(VPMM_PwrSta_enum)
  VINP_IVINightModeSta_flg/1 -> [VINP_IVINightModeSta_flg]
  [VINP_IVINightModeSta_flg] -> Dimmer/3(VINP_IVINightModeSta_flg)
  [VBCM_AntitheftSta_enum] -> VBCM_AntitheftSta_enum/1
  [VBCM_HornCtrl_flg] -> VBCM_HornCtrl_flg/1
  [VBCM_AllDoorSW_flg] -> VBCM_AllDoorSW_flg/1
  [VBCM_BCMDoorLockSta_flg] -> VBCM_BCMDoorLockSta_flg/1
  [VBCM_HoodSW_flg] -> VBCM_HoodSW_flg/1
  [VBCM_TailgateSW_flg] -> VBCM_TailgateSW_flg/1
  [VINP_CANMsgValidIVI2_flg] -> Dimmer/5(VINP_CANMsgValidIVI2_flg)
  VINP_ReOutsideMirror_enum/1 -> PowerMirror/5(VINP_ReOutsideMirror_enum)
  BCM_WAKE_MODULE/2(VBCM_WakeUp_flg) -> [VBCM_WakeUp_flg]
  [VPMM_PwrSta_enum] -> Amb/5(VPMM_PwrSta_enum)
  [VBCM_PosLamp_flg] -> Amb/6(VBCM_PosLamp_flg)
  [VBCM_WakeUp_flg] -> Amb/7(VBCM_WakeUp_flg)
  Amb/2(VBCM_AmbLightBreath1_enum) -> VBCM_AmbLightBreath1_enum/1
  Amb/3(VBCM_AmbLightBreath2_enum) -> VBCM_AmbLightBreath2_enum/1
  Amb/4(VBCM_AmbLightBreath3_enum) -> VBCM_AmbLightBreath3_enum/1
  Amb/8(VBCM_AmbLightBrightness1_enum) -> VBCM_AmbLightBrightness1_enum/1
  Amb/9(VBCM_AmbLightBrightness2_enum) -> VBCM_AmbLightBrightness2_enum/1
  Amb/10(VBCM_AmbLightBrightness3_enum) -> VBCM_AmbLightBrightness3_enum/1
  Amb/14(VBCM_AmbLightColor1_enum) -> VBCM_AmbLightColor1_enum/1
  Amb/15(VBCM_AmbLightColor2_enum) -> VBCM_AmbLightColor2_enum/1
  Amb/16(VBCM_AmbLightColor3_enum) -> VBCM_AmbLightColor3_enum/1
  Amb/1(VBCM_LampPwr_flg) -> VBCM_LampPwr_flg/1
  VINP_IVIPWModeReq_enum/1 -> Amb/2(VINP_IVIPWModeReq_enum)
  [VINP_IVINightModeSta_flg] -> Amb/3(VINP_IVINightModeSta_flg)
  VINP_FlashAntitheft_enum/1 -> Verify/1(VINP_FlashAntitheft_enum)
  Verify/1(VBCM_FlashAntitheft_enum) -> AntiTheft/13(VBCM_FlashAntitheft_enum), [VBCM_FlashAntitheft_enum]  "VBCM_FlashAntitheft_enum"
  [VPMM_PwrSta_enum] -> WasherWiper/8(VPMM_PwrSta_enum)
  [VINP_CANMsgValidIVI2_flg] -> WasherWiper/10(VINP_CANMsgValidIVI2_flg)
  VINP_FWiperProtection_flg/1 -> WasherWiper/12(VINP_FWiperProtection_flg)
  VINP_RLSRainSnrWiperCmd_enum/1 -> WasherWiper/3(VINP_RLSRainSnrWiperCmd_enum)
  VINP_FWiperAS_flg/1 -> WasherWiper/4(VINP_FWiperAS_flg)
  VINP_RWiperAS_flg/1 -> WasherWiper/6(VINP_RWiperAS_flg)
  VINP_IVIWIMAINSW_flg/1 -> WasherWiper/9(VINP_IVIWIMAINSW_flg)
  VINP_RWiperProtection_flg/1 -> WasherWiper/11(VINP_RWiperProtection_flg)
  WasherWiper/1(VBCM_FrWiperL_flg) -> VBCM_FWiperL_flg/1
  WasherWiper/2(VBCM_FrWiperH_flg) -> VBCM_FWiperH_flg/1
  WasherWiper/3(VBCM_RrWiper_flg) -> VBCM_RWiper_flg/1
  WasherWiper/4(VBCM_WasherCtrl_enum) -> VBCM_WasherCtrl_enum/1
  WasherWiper/5(VBCM_WiperFixMode_flg) -> VBCM_WiperFixMode_flg/1
  PTG/2(VBCM_APSOpenPTG_flg) -> [VBCM_APSOpenPTG_flg]  "VBCM_APSOpenPTG_flg"
  [VTQD_ShiftGearPosn_enum] -> PTG/7(VTQD_ShiftGearPosn_enum)
  [VPMM_PwrSta_enum] -> PTG/6(VPMM_PwrSta_eunm)
  [VINP_VehSpeed_kph] -> PTG/10(VINP_VehSpeed_kph)
  PTG/1(VBCM_SPTGDet_flg) -> [VBCM_SPTGDet_flg]  "VBCM_SPTGDet_flg"
  VAPM_PASDRMR_cm/1 -> PTG/3(VAPM_PASDRMR_cm)
  VAPM_PASDRML_cm/1 -> PTG/4(VAPM_PASDRML_cm)
  [VINP_CANMsgValidIVI2_flg] -> PTG/9(VINP_CANMsgValidIVI2_flg)
  [VINP_PCommandToBCM_enum] -> PTG/5(VINP_PCommandToBCM_enum)
  [VINP_TailgateSW_flg] -> PTG/2(VINP_TailgateSW_flg)
  VINP_PDKeyAreaPTG_enum/1 -> PTG/1(VINP_PDKeyAreaPTG_enum)
  VINP_IVIPTGUSStaSW_flg/1 -> PTG/8(VINP_IVIPTGUSStaSW_flg)
  [VBCM_APSOpenPTG_flg] -> AntiTheft/14(VINP_APSOpenPTG_flg)
  [VBCM_SPTGDet_flg] -> FlasherSignal/14(VINP_SPTGDet_flg)
  VTQD_ShiftGearPosn_enum/1 -> [VTQD_ShiftGearPosn_enum]
  [VTQD_ShiftGearPosn_enum] -> ExteriorLight/8(VTQD_ShiftGearPosn_enum)
  VINP_PCommandToBCM_enum/1 -> [VINP_PCommandToBCM_enum]
  [VINP_PCommandToBCM_enum] -> AntiTheft/1(VINP_PCommandToBCM_enum)
  Constant8/1 -> IVI Reset/2(KBCM_IVIRstHoldT_ms)
  Constant9/1 -> IVI Reset/3(KBCM_IVIRstTriggerT_ms)
  VINP_SWCmodeSta_flg/1 -> IVI Reset/1(VINP_SWCmodeSta_flg)
  IVI Reset/1(VBCM_IVIRST_flg) -> VBCM_IVIRST_flg/1
  [VBCM_APSOpenPTG_flg] -> VBCM_APSOpenPTG_flg/1
  [VBCM_SPTGDet_flg] -> VBCM_SPTGDet_flg/1
  [VBCM_PosLamp_flg] -> VBCM_PosLamp_flg/1
  ExteriorLight/11(VBCM_FollowMe_flg) -> VBCM_FollowMe_flg/1
  [VBCM_LBSD_flg] -> VBCM_LBSD_flg/1
  [VBCM_RBSD_flg] -> VBCM_RBSD_flg/1
  [VBCM_LTurnLP_flg] -> VBCM_LTurnLP_flg/1
  [VBCM_RTurnLP_flg] -> VBCM_RTurnLP_flg/1
  VDDM_MCUActCFS_flg/1 -> FlasherSignal/21(VDDM_MCUActCFS_flg)
  VDDM_HVRlyOpCFS_flg/1 -> FlasherSignal/20(VDDM_HVRlyOpCFS_flg)
  Constant14/1 -> RoomLamp/13(KBCM_RmLampKeep_min)
  VINP_FlashMFSWTri_flg/1 -> PowerMirror/6(EEP_MFSWTri_flg)
  VINP_FlashMirrorFlodPos/1 -> PowerMirror/7(EEP_MirrorFlodPos)
  PowerMirror/2(MFSWTri) -> VBCM_MFSWTri_flg/1
  PowerMirror/3(MirrorFlodPos) -> VBCM_MirrorFlodPos_flg/1
  VINP_FlashFuelDoorPos/1 -> CenterDoorLock/16(EEP_FuelDoorPos)
  CenterDoorLock/9(VBCM_FuelDoorPos_flg) -> VBCM_FuelDoorPos_flg/1
  VINP_FlashCountAlarm_enum/1 -> AntiTheft/15(VINP_FlashCountAlarm_enum)
  AntiTheft/16(VBCM_CountAlarm_enum) -> VBCM_CountAlarm_enum/1
  Constant10/1 -> PTG/12(KBCM_DelayTSW_flg)
  Constant11/1 -> PTG/13(KBCM_ReDetectT_K)
  Constant12/1 -> PTG/14(KBCM_SPTGDetectT_sec)
  Constant13/1 -> PTG/15(KBCM_SPTGLeave_flg)
  Constant15/1 -> PTG/16(KBCM_SPTGWaitDKC_sec)
  VINP_CANMsgValidDKC1_flg/1 -> PTG/11(VINP_CANMsgValidDKC1_flg)
  VINP_FlashLockSetting_flg/1 -> CenterDoorLock/17(EEP_LockSetting)
  VINP_FlashMFRDNBrightReq_pct/1 -> Dimmer/6(EEP_MFRDNBrightReq)
  VINP_FlashRoomLampMode_flg/1 -> RoomLamp/14(EEP_RoomLampMode)
  VINP_FlashWiperFixMode_flg/1 -> WasherWiper/13(VINP_FlashWiperFixMode)
  Dimmer/3(VBCM_MFRDNBrightReq_pct) -> VBCM_MFRDNBrightReq_pct/1
  Sum/1 -> Unit Delay1/1
  Switch/1 -> Sum/2
  Constant17/1 -> Switch/3
  Constant16/1 -> Switch/1
  Unit Delay1/1 -> [BCMInitial], Switch/2, Sum/1
  [BCMInitial] -> WasherWiper/14(BCMInitial)
  [BCMInitial] -> RoomLamp/15(BCMInitial)
  [BCMInitial] -> Dimmer/7(BCMInitial)
  [BCMInitial] -> PTG/18(BCMInitial)
  VINP_FlashIVIPTGUSStaSW_flg/1 -> PTG/17(EEP_IVIPTGUSStaSW)
  PTG/3(VBCM_IVIPTGUSStaSW_flg) -> VBCM_IVIPTGUSStaSW_flg/1
  Data Type Conversion/1 -> VBCM_PTGInnerSW2_enum/1  "VBCM_PTGInnerSW2_enum"
  VINP_PTGInnerSW2_enum/1 -> Data Type Conversion/1
  VINP_FlashHoodSW_flg/1 -> [VINP_FlashHoodSW_flg]
  VINP_FlashTailgateSW_flg/1 -> [VINP_FlashTailgateSW_flg]
  VINP_FlashCTDLockSW_flg/1 -> [VINP_FlashCTDLockSW_flg]
  VINP_FlashTailgateHDSW_flg/1 -> [VINP_FlashTailgateHDSW_flg]
  [VINP_FlashHoodSW_flg] -> BCM_WAKE_MODULE/18(VINP_FlashHoodSW_flg)
  [VINP_FlashTailgateSW_flg] -> BCM_WAKE_MODULE/19(VINP_FlashTailgateSW_flg)
  [VINP_FlashCTDLockSW_flg] -> BCM_WAKE_MODULE/20(VINP_FlashCTDLockSW_flg)
  [VINP_FlashTailgateHDSW_flg] -> BCM_WAKE_MODULE/21(VINP_FlashTailgateHDSW_flg)
  [VINP_CANMsgValidGWZoneDR1_flg] -> APM_Door/18(VINP_CANMsgValidGWZoneDR1_flg)
  [VINP_CANMsgValidGWZoneFR1_flg] -> APM_Door/19(VINP_CANMsgValidGWZoneFR1_flg)
  APM_Door/4(VBCM_LRRDCtrlCmd_pct) -> VBCM_LRRDCtrlCmd_pct/1
  APM_Door/2(VBCM_LPasCtrlCmd_pct) -> VBCM_LPasCtrlCmd_pct/1
  APM_Door/3(VBCM_LRLDCtrlCmd_pct) -> VBCM_LRLDCtrlCmd_pct/1
  [VINP_RLDoorSW_flg] -> APM_Door/11(VINP_RLDoorSW_flg)
  [VINP_DrDoorSW_flg] -> APM_Door/5(VINP_DrDoorSW_flg)
  APM_Door/5(VBCM_APMDoorControlSta_flg) -> VBCM_APMDoorControlSta_flg/1
  VINP_LRRDValWdwOpened_pct/1 -> APM_Door/13(VINP_LRRDValWdwOpened_pct)
  [VINP_CANMsgValidIVI2_flg] -> APM_Door/17(VINP_CANMsgValidIVI2_flg)
  [task_time_s] -> APM_Door/1(task_time_s)
  VINP_FlashAPMDoorControlSta_flg/1 -> APM_Door/15(VINP_FlashAPMDoorControlSta_flg)
  VINP_LPasControlCommand_pct/1 -> APM_Door/6(VINP_LPasControlCommand_pct)
  VINP_OpenDrOpenWdoSW_flg/1 -> APM_Door/2(VINP_OpenDrOpenWdoSW_flg)
  VINP_LDrvValWdwOpened_pct/1 -> APM_Door/4(VINP_LDrvValWdwOpened_pct)
  VINP_LPasValWdwOpened_pct/1 -> APM_Door/7(VINP_LPasValWdwOpened_pct)
  VINP_LRLDControlCommand_pct/1 -> APM_Door/9(VINP_LRLDControlCommand_pct)
  VINP_LRRDControlCommand_pct/1 -> APM_Door/12(VINP_LRRDControlCommand_pct)
  APM_Door/1(VBCM_LDrvCtrlCmd_pct) -> VBCM_LDrvCtrlCmd_pct/1
  [VINP_RRDoorSW_flg] -> APM_Door/14(VINP_RRDoorSW_flg)
  [VINP_PsDoorSW_flg] -> APM_Door/8(VINP_PsDoorSW_flg)
  VINP_LRLDValWdwOpened_pct/1 -> APM_Door/10(VINP_LRLDValWdwOpened_pct)
  [BCMInitial] -> APM_Door/16(BCMInitial)
  VINP_LDrvControlCommand_pct/1 -> APM_Door/3(VINP_LDrvControlCommand_pct)
  VINP_PsDoorSW_flg/1 -> [VINP_PsDoorSW_flg]
  VINP_RLDoorSW_flg/1 -> [VINP_RLDoorSW_flg]
  VINP_RRDoorSW_flg/1 -> [VINP_RRDoorSW_flg]
  [VINP_PsDoorSW_flg] -> AntiTheft/6(VINP_PsDoorSW_flg)
  [VINP_RLDoorSW_flg] -> AntiTheft/7(VINP_RLDoorSW_flg)
  [VINP_RRDoorSW_flg] -> AntiTheft/8(VINP_RRDoorSW_flg)
  VINP_CANMsgValidGWZoneDR1_flg/1 -> [VINP_CANMsgValidGWZoneDR1_flg]
  VINP_CANMsgValidGWZoneFR1_flg/1 -> [VINP_CANMsgValidGWZoneFR1_flg]
  [VINP_CANMsgValidGWZoneFR1_flg] -> AntiTheft/17(VINP_CANMsgValidGWZoneFR1_flg)
  [VINP_CANMsgValidGWZoneDR1_flg] -> AntiTheft/16(VINP_CANMsgValidGWZoneDR1_flg)
  RoomLamp/1(VBCM_RoomLampH_flg) -> [VBCM_RoomLampH_flg], VBCM_RoomLampH_flg/1
  RoomLamp/2(VBCM_RoomLampL_flg) -> VBCM_RoomLampL_flg/1
  RoomLamp/3(VBCM_RoomLampMode_flg) -> VBCM_RoomLampMode_flg/1
  [task_time_s] -> RoomLamp/1(task_time_s)
  [VINP_DrDoorSW_flg] -> RoomLamp/6(VINP_DrDoorSW_flg)
  [VINP_PsDoorSW_flg] -> RoomLamp/7(VINP_PsDoorSW_flg)
  [VINP_RLDoorSW_flg] -> RoomLamp/8(VINP_RLDoorSW_flg)
  [VINP_RRDoorSW_flg] -> RoomLamp/9(VINP_RRDoorSW_flg)
  Constant18/1 -> RoomLamp/18(KBCM_RmLpKeyInT_s)  "2400"
  VINP_PDKeyAreaLockUnlock_enum/1 -> RoomLamp/16(VINP_PDKeyAreaLockUnlock_enum)
  Constant19/1 -> RoomLamp/19(KBCM_RmLpKeyMissT_s)  "600"
  VINP_PDKeyAreaPS_enum/1 -> RoomLamp/17(VINP_PDKeyAreaPS_enum)
  VINP_DiagFLTC_mA/1 -> [VINP_DiagFLTC_mA]
  VINP_DiagFRTC_mA/1 -> [VINP_DiagFRTC_mA]
  VINP_DiagRLTC_mA/1 -> [VINP_DiagRLTC_mA]
  VINP_DiagRRTC_mA/1 -> [VINP_DiagRRTC_mA]
  VINP_funAuto_flg/1 -> [VINP_funAuto_flg]
  VINP_DiagDRLOFF_flg/1 -> [VINP_DiagDRLOFF_flg]
  VINP_DiagFMHT_s/1 -> [VINP_DiagFMHT_s]
  [VINP_funAuto_flg] -> CenterDoorLock/11(VINP_funAuto_flg)
  [VINP_DiagDRLOFF_flg] -> ExteriorLight/22(VINP_DiagDRLOFF_flg)
  [task_time_s] -> ExteriorLight/1(task_time_s)
  Constant45/1 -> Add1/2
  Gain1/1 -> Add1/1
  Add1/1 -> ExteriorLight/23(VINP_DiagFMHT_s)
  Constant44/1 -> Gain1/1
  [VINP_DiagFMHT_s] -> Terminator/1
  Constant49/1 -> Gain4/1
  Constant48/1 -> Gain3/1
  Constant47/1 -> Gain2/1
  Constant46/1 -> Gain/1
  Gain/1 -> FlasherSignal/16(VBCM_DiagFLTC_mA)
  Gain2/1 -> FlasherSignal/17(VBCM_DiagFRTC_mA)
  Gain3/1 -> FlasherSignal/18(VBCM_DiagRLTC_mA)
  Gain4/1 -> FlasherSignal/19(VBCM_DiagRRTC_mA)
  [VINP_DiagFLTC_mA] -> Terminator1/1
  [VINP_DiagFRTC_mA] -> Terminator2/1
  [VINP_DiagRLTC_mA] -> Terminator3/1
  [VINP_DiagRRTC_mA] -> Terminator4/1
  FlasherSignal/3(VBCM_RTurnLP_flg) -> [VBCM_RTurnLP_flg]
  FlasherSignal/4(VBCM_OutMode_enum) -> [VBCM_OutMode_enum]
  FlasherSignal/5(VBCM_BCMBuzzerReq_flg) -> VBCM_BCMBuzzerReq_flg/1
  FlasherSignal/6(VBCM_DiagFLTS_flg) -> VBCM_DiagFLTS_flg/1
  FlasherSignal/7(VBCM_DiagFRTS_flg) -> VBCM_DiagFRTS_flg/1
  FlasherSignal/8(VBCM_DiagRLTS_flg) -> VBCM_DiagRLTS_flg/1
  FlasherSignal/9(VBCM_DiagRRTS_flg) -> VBCM_DiagRRTS_flg/1
  VINP_APSActive_flg/1 -> FlasherSignal/22(VINP_APSActive_flg)
  VINP_AVMparkingmode_enum/1 -> FlasherSignal/23(VINP_AVMparkingmode_enum)
  [task_time_s] -> FlasherSignal/24(task_time_s)
  [task_time_s] -> Amb/1(task_time_s)
  [VBCM_AllDoorSW_flg] -> Amb/4(VBCM_AllDoorSW_flg)
  [VBCM_AntitheftSta_enum] -> Amb/20(AntitheftSta)
  [VBCM_FlashAntitheft_enum] -> Amb/21(EEP_AntitheftSta)
  VINP_HVBattSOCDis_pct/1 -> Amb/22(VINP_HVBattSOCDis_pct)
  Amb/5(VBCM_AmbLightBreath4_enum) -> VBCM_AmbLightBreath4_enum/1
  Amb/6(VBCM_AmbLightBreath5_enum) -> VBCM_AmbLightBreath5_enum/1
  Amb/7(VBCM_AmbLightBreath6_enum) -> VBCM_AmbLightBreath6_enum/1
  Amb/11(VBCM_AmbLightBrightness4_enum) -> VBCM_AmbLightBrightness4_enum/1
  Amb/12(VBCM_AmbLightBrightness5_enum) -> VBCM_AmbLightBrightness5_enum/1
  Amb/13(VBCM_AmbLightBrightness6_enum) -> VBCM_AmbLightBrightness6_enum/1
  Amb/17(VBCM_AmbLightColor4_enum) -> VBCM_AmbLightColor4_enum/1
  Amb/18(VBCM_AmbLightColor5_enum) -> VBCM_AmbLightColor5_enum/1
  Amb/19(VBCM_AmbLightColor6_enum) -> VBCM_AmbLightColor6_enum/1
  VINP_SRRBSDWarnL_enum/1 -> [VINP_SRRBSDWarnL_enum]
  [VINP_SRRODAWarnL_enum] -> Amb/8(VINP_SRRODAWarnL_enum)
  [VINP_SRRODAWarnR_enum] -> Amb/9(VINP_SRRODAWarnR_enum)
  [VINP_SRRBSDWarnL_enum] -> Amb/10(VINP_SRRBSDWarnL_enum)
  [VINP_SRRBSDWarnR_enum] -> Amb/11(VINP_SRRBSDWarnR_enum)
  [FDC_BCM_AmbPwrWarnEN_Sta] -> Amb/16(VINP_AmbPwrWarnEN_flg)
  [FDC_BCM_AmbLinkDriSta_Sta] -> Amb/19(VINP_AmbLinkDriSta_flg)
  [FDC_BCM_AmbBrightSta_Sta] -> Amb/17(VINP_AmbBrightnessSta_enum)
  [FDC_BCM_AmbColorSta_Sta] -> Amb/18(VINP_AmbColorSta_enum)
  [FDC_BCM_AmbODAEN_Sta] -> Amb/15(VINP_AmbODAEN_flg)
  [FDC_BCM_AmbFunEN_Sta] -> Amb/12(VINP_AmbFunEN_flg)
  [FDC_BCM_AmbWelEN_Sta] -> Amb/13(VINP_AmbWelEN_flg)
  [FDC_BCM_AmbDimEN_Sta] -> Amb/14(VINP_AmbDimEN_flg)
  VINP_IVILockSoundSWSta_flg/1 -> AntiTheft/19(VINP_IVILockSoundSWSta_flg)
  AntiTheft/17(VBCM_LockAlarm_enum) -> VBCM_LockAlarm_enum/1
  CenterDoorLock/11(VBCM_fUnlockSingle_flg) -> VBCM_fUnlockSingle_flg/1
  VINP_FlashfUnlockSingle_flg/1 -> CenterDoorLock/18(VINP_FlashfUnlockSingle_flg)
  [VINP_SRRODAWarnR_enum] -> ExteriorLight/14(VINP_SRRODAWarnR_flg)
  [VINP_SRRODAWarnL_enum] -> ExteriorLight/15(VINP_SRRODAWarnL_flg)
  [VINP_SRRBSDWarnL_enum] -> ExteriorLight/17(VINP_SRRBSDWarnL_flg)
  [VINP_SRRBSDWarnR_enum] -> ExteriorLight/16(VINP_SRRBSDWarnR_flg)
  [VBCM_ATCtrl_enum] -> VBCM_ATCtrl_enum/1
  VINP_AmbLightSW_flg/1 -> Personal_Setting/3(VINP_AmbLightSW_flg)
  VINP_AmbLightWlcmLightSW_flg/1 -> Personal_Setting/5(VINP_AmbLightWlcmLightSW_flg)
  VINP_AmbLightDimInDarkSW_flg/1 -> Personal_Setting/7(VINP_AmbLightDimInDarkSW_flg)
  VINP_LINKtoDRIVE_flg/1 -> Personal_Setting/9(VINP_LINKtoDRIVE_flg)
  VINP_AmbLighLowBatAlertSW_flg/1 -> Personal_Setting/11(VINP_AmbLighLowBatAlertSW_flg)
  VINP_AmbLighSafetyAlertSW_flg/1 -> Personal_Setting/13(VINP_AmbLighSafetyAlertSW_flg)
  VINP_AmbLightBrightnessSet_enum/1 -> Personal_Setting/22(VINP_AmbLightBrightnessSet_enum)
  VINP_AmbLightColorSet_enum/1 -> Personal_Setting/15(VINP_AmbLightColorSet_enum)
  [FDC_BCM_AmbFunEN_Sta] -> VBCM_AmbFunEN_flg/1
  [FDC_BCM_AmbWelEN_Sta] -> VBCM_AmbWelEN_flg/1
  [FDC_BCM_AmbDimEN_Sta] -> VBCM_AmbDimEN_flg/1
  [FDC_BCM_AmbLinkDriSta_Sta] -> VBCM_AmbLinkDriSta_flg/1
  [FDC_BCM_AmbPwrWarnEN_Sta] -> VBCM_AmbPwrWarnEN_flg/1
  [FDC_BCM_AmbODAEN_Sta] -> VBCM_AmbODAEN_flg/1
  [FDC_BCM_AmbColorSta_Sta] -> VBCM_AmbColorSta_enum/1
  [FDC_BCM_AmbBrightSta_Sta] -> VBCM_AmbBrightSta_enum/1
  VINP_FlashAmbColorSta5_enum/1 -> Personal_Setting/20(VINP_FlashAmbColorSta5_enum)
  VINP_FlashAmbColorSta7_enum/1 -> Personal_Setting/21(VINP_FlashAmbColorSta7_enum)
  VINP_FlashAmbBrightnessSta5_enum/1 -> Personal_Setting/27(VINP_FlashAmbBrightnessSta5_enum)
  VINP_FlashAmbBrightnessSta7_enum/1 -> Personal_Setting/28(VINP_FlashAmbBrightnessSta7_enum)
  VINP_FlashAmbColorSta1_enum/1 -> Personal_Setting/16(VINP_FlashAmbColorSta1_enum)
  VINP_FlashAmbColorSta2_enum/1 -> Personal_Setting/17(VINP_FlashAmbColorSta2_enum)
  VINP_FlashAmbColorSta3_enum/1 -> Personal_Setting/18(VINP_FlashAmbColorSta3_enum)
  VINP_FlashAmbColorSta4_enum/1 -> Personal_Setting/19(VINP_FlashAmbColorSta4_enum)
  VINP_FlashAmbBrightnessSta1_enum/1 -> Personal_Setting/23(VINP_FlashAmbBrightnessSta1_enum)
  VINP_FlashAmbBrightnessSta2_enum/1 -> Personal_Setting/24(VINP_FlashAmbBrightnessSta2_enum)
  VINP_FlashAmbBrightnessSta3_enum/1 -> Personal_Setting/25(VINP_FlashAmbBrightnessSta3_enum)
  VINP_FlashAmbBrightnessSta4_enum/1 -> Personal_Setting/26(VINP_FlashAmbBrightnessSta4_enum)
  VINP_FlashAmbDimEN_enum/1 -> Personal_Setting/8(VINP_FlashAmbDimEN_enum)
  VINP_FlashAmbLinkDriSta_enum/1 -> Personal_Setting/10(VINP_FlashAmbLinkDriSta_enum)
  VINP_FlashAmbPwrWarnEN_enum/1 -> Personal_Setting/12(VINP_FlashAmbPwrWarnEN_enum)
  VINP_FlashAmbODAEN_enum/1 -> Personal_Setting/14(VINP_FlashAmbODAEN_enum)
  VINP_FlashAmbFunEN_enum/1 -> Personal_Setting/4(VINP_FlashAmbFunEN_enum)
  VINP_FlashAmbWelEN_enum/1 -> Personal_Setting/6(VINP_FlashAmbWelEN_enum)
  VINP_UserSet_enum/1 -> Personal_Setting/1(UserNow)
  VINP_CANMsgValidIVI1_flg/1 -> [VINP_CANMsgValidIVI1_flg]
  [VINP_CANMsgValidIVI1_flg] -> AntiTheft/18(VINP_CANMsgValidIVI1_flg)
  [VINP_CANMsgValidIVI1_flg] -> Personal_Setting/2(VINP_CANMsgValidIVI1_flg)
  Personal_Setting/21(FDC_BCM_AmbBrightSta_Sta) -> [FDC_BCM_AmbBrightSta_Sta]  "VBCM_AmbBrightSta_enum"
  Personal_Setting/14(FDC_BCM_AmbColorSta_Sta) -> [FDC_BCM_AmbColorSta_Sta]  "VBCM_AmbColorSta_enum"
  Personal_Setting/10(FDC_BCM_AmbPwrWarnEN_Sta) -> [FDC_BCM_AmbPwrWarnEN_Sta]  "VBCM_AmbPwrWarnEN_flg"
  Personal_Setting/12(FDC_BCM_AmbODAEN_Sta) -> [FDC_BCM_AmbODAEN_Sta]  "VBCM_AmbODAEN_flg"
  Personal_Setting/8(FDC_BCM_AmbLinkDriSta_Sta) -> [FDC_BCM_AmbLinkDriSta_Sta]  "VBCM_AmbLinkDriSta_flg"
  Personal_Setting/1(VBCM_UserNow_enum) -> VBCM_UserNow_enum/1  "VBCM_UserNow_enum"
  Personal_Setting/22(VBCM_AmbBrightnessSta1_enum) -> VBCM_AmbBrightnessSta1_enum/1  "VBCM_AmbBrightnessSta1_enum"
  Personal_Setting/6(FDC_BCM_AmbDimEN_Sta) -> [FDC_BCM_AmbDimEN_Sta]  "VBCM_AmbDimEN_flg"
  Personal_Setting/23(VBCM_AmbBrightnessSta2_enum) -> VBCM_AmbBrightnessSta2_enum/1  "VBCM_AmbBrightnessSta2_enum"
  Personal_Setting/20(VBCM_AmbColorSta7_enum) -> VBCM_AmbColorSta7_enum/1  "VBCM_AmbColorSta7_enum"
  Personal_Setting/24(VBCM_AmbBrightnessSta3_enum) -> VBCM_AmbBrightnessSta3_enum/1  "VBCM_AmbBrightnessSta3_enum"
  Personal_Setting/4(FDC_BCM_AmbWelEN_Sta) -> [FDC_BCM_AmbWelEN_Sta]  "VBCM_AmbWelEN_flg"
  Personal_Setting/19(VBCM_AmbColorSta5_enum) -> VBCM_AmbColorSta5_enum/1  "VBCM_AmbColorSta5_enum"
  Personal_Setting/25(VBCM_AmbBrightnessSta4_enum) -> VBCM_AmbBrightnessSta4_enum/1  "VBCM_AmbBrightnessSta4_enum"
  Personal_Setting/18(VBCM_AmbColorSta4_enum) -> VBCM_AmbColorSta4_enum/1  "VBCM_AmbColorSta4_enum"
  Personal_Setting/26(VBCM_AmbBrightnessSta5_enum) -> VBCM_AmbBrightnessSta5_enum/1  "VBCM_AmbBrightnessSta5_enum"
  Personal_Setting/2(FDC_BCM_AmbFunEN_Sta) -> [FDC_BCM_AmbFunEN_Sta]  "VBCM_AmbFunEN_flg"
  Personal_Setting/17(VBCM_AmbColorSta3_enum) -> VBCM_AmbColorSta3_enum/1  "VBCM_AmbColorSta3_enum"
  Personal_Setting/27(VBCM_AmbBrightnessSta7_enum) -> VBCM_AmbBrightnessSta7_enum/1  "VBCM_AmbBrightnessSta7_enum"
  Personal_Setting/16(VBCM_AmbColorSta2_enum) -> VBCM_AmbColorSta2_enum/1  "VBCM_AmbColorSta2_enum"
  Personal_Setting/15(VBCM_AmbColorSta1_enum) -> VBCM_AmbColorSta1_enum/1  "VBCM_AmbColorSta1_enum"
  Personal_Setting/13(VBCM_AmbODAENMem_enum) -> VBCM_AmbODAENFlash_enum/1  "VBCM_AmbODAENFlash_enum"
  Personal_Setting/11(VBCM_AmbPwrWarnENMem_enum) -> VBCM_AmbPwrWarnENFlash_enum/1  "VBCM_AmbPwrWarnENFlash_enum"
  Personal_Setting/9(VBCM_AmbLinkDriStaMem_enum) -> VBCM_AmbLinkDriStaFlash_enum/1  "VBCM_AmbLinkDriStaFlash_enum"
  Personal_Setting/7(VBCM_AmbDimENMem_enum) -> VBCM_AmbDimENFlash_enum/1  "VBCM_AmbDimENFlash_enum"
  Personal_Setting/5(VBCM_AmbWelENMem_enum) -> VBCM_AmbWelENFlash_enum/1  "VBCM_AmbWelENFlash_enum"
  Personal_Setting/3(VBCM_AmbFunENMem_enum) -> VBCM_AmbFunENFlash_enum/1  "VBCM_AmbFunENFlash_enum"
  FlasherSignal/10(VBCM_HazardIND_flg) -> VBCM_HazardIND_flg/1
  [VBCM_DimSwSta_flg] -> VBCM_DimSwSta_flg/1  "VBCM_DimSwSta_flg"
  [VBCM_TurnSwSta_enum] -> VBCM_TurnSwSta_enum/1  "VBCM_TurnSwSta_enum"
  [VBCM_FWasSwSta_enum] -> VBCM_FWasSwSta_enum/1  "VBCM_FWasSwSta_enum"
  [VBCM_FWipSwSta_enum] -> VBCM_FWipSwSta_enum/1  "VBCM_FWipSwSta_enum"
  [VBCM_PassSWSta_flg] -> VBCM_PassSWSta_flg/1  "VBCM_PassSWSta_flg"
  VINP_SASAngle_Deg/1 -> CSW/12(VINP_SASAngle_deg)
  VINP_TurnSwTimeSet_enum/1 -> CSW/13(VINP_TurnSwTimeSet_enum)
  VINP_CSW2FWasSwSta_enum/1 -> CSW/11(VINP_CSW2FWasSwSta_enum)
  VINP_CSW2FWipSwSta_enum/1 -> CSW/9(VINP_CSW2FWipSwSta_enum)
  VINP_CSW2RWipWasSwSta_enum/1 -> CSW/15(VINP_CSW2RWIPWasSwSta_enum)
  VINP_CSW2DimSwSta_flg/1 -> CSW/3(VINP_CSW2DimSwSta_flg)
  VINP_CSW2PassSWSta_flg/1 -> CSW/5(VINP_CSW2PassSWSta_flg)
  VUNP_CSW2TurnSwSta_enum/1 -> CSW/7(VINP_CSW2TurnSwSta_enum)
  [task_time_s] -> CSW/1(task_time_s)
  ExteriorLight/2(VBCM_LBeam_flg) -> [VBCM_LBeam_flg]
  [VBCM_LBeam_flg] -> VBCM_LBeam_flg/1
  Unit Delay2/1 -> CSW/14(VINP_LBeam_flg)
  [VBCM_LBeam_flg] -> Unit Delay2/1
  VINP_CSWTurnSWSta_enum/1 -> [VINP_CSWTurnSWSta_enum]
  [VINP_CSWTurnSWSta_enum] -> CSW/6(VINP_CSWTurnSwSta_enum)
  VINP_CSWDimSw_flg/1 -> [VINP_CSWDimSw_flg]
  VINP_CSWPassSWSta_flg/1 -> [VINP_CSWPassSWSta_flg]
  [VINP_CSWDimSw_flg] -> CSW/2(VINP_CSWDimSwSta_flg)
  [VINP_CSWPassSWSta_flg] -> CSW/4(VINP_CSWPassSWSta_flg)
  VINP_CSWFWasSWSta_enum/1 -> [VINP_CSWFWasSWSta_enum]
  VINP_CSWRWasSWSta_enum/1 -> [VINP_CSWRWasSWSta_enum]
  VINP_CSWRWipIntSwSta_enum/1 -> [VINP_CSWRWipIntSwSta_enum]
  VINP_CSWFWipSWSta_enum/1 -> [VINP_CSWFWipSWSta_enum]
  [VINP_CSWFWipSWSta_enum] -> CSW/8(VINP_CSWFWipSwSta_enum)
  [VINP_CSWFWasSWSta_enum] -> CSW/10(VINP_CSWFWasSwSta_enum)
  [VINP_CSWRWipIntSwSta_enum] -> CSW/16(VINP_CSWRWipIntSwSta_enum)
  [VINP_CSWRWasSWSta_enum] -> CSW/17(VINP_CSWRWasSWSta_enum)
  CSW/4(VBCM_FWipSwSta_enum) -> [VBCM_FWipSwSta_enum]
  CSW/5(VBCM_FWasSwSta_enum) -> [VBCM_FWasSwSta_enum]
  CSW/6(VBCM_RWasSwSta_enum) -> [VBCM_RWasSwSta_enum]
  CSW/1(VBCM_DimSwSta_flg) -> [VBCM_DimSwSta_flg]
  CSW/2(VBCM_PassSWSta_flg) -> [VBCM_PassSWSta_flg]
  CSW/3(VBCM_TurnSwSta_enum) -> [VBCM_TurnSwSta_enum]
  CSW/7(VBCM_RWipIntSwSta_enum) -> [VBCM_RWipIntSwSta_enum]
  [VBCM_FWasSwSta_enum] -> WasherWiper/1(VINP_CSWFWasSWSta_enum)
  [VBCM_RWipIntSwSta_enum] -> WasherWiper/5(VINP_CSWRWipIntSwSta_enum)
  [VBCM_FWipSwSta_enum] -> WasherWiper/2(VINP_CSWFWipSWSta_enum)
  [VBCM_RWasSwSta_enum] -> WasherWiper/7(VINP_CSWRWasSWSta_enum)
  [VBCM_TurnSwSta_enum] -> FlasherSignal/5(VINP_CSWTurnSWSta_enum)
  [VBCM_PassSWSta_flg] -> ExteriorLight/7(VINP_CSWPassSWSta_flg)
  [VBCM_DimSwSta_flg] -> ExteriorLight/6(VINP_CSWDimSw_flg)
